simulink model "double_sim_motor"  (R2022b)
settings: Solver=FixedStepAuto  StartTime=0.0  StopTime=T-0.1  RelTol=1e-3
values from neighbouring files (symbols this model uses):
  dt = 0.005    [double_main.m]    (also in double_main_px4.m; double_main_so3.m; se3controller.m = 0.001)
  f1234tofm = [1 1 1 1 ... (first row only)    [double_main.m]    (also in double_main_px4.m; double_main_so3.m; my_exp1.m)
  fmtof1234 = inv(f1234tofm)    [double_main.m]    (also in double_main_px4.m; double_main_so3.m; my_exp1.m)
  J = diag([0.0024 0.0025 0.0041])    [double_main.m]    (also in double_main_px4.m = diag([0.0031 0.0032 0.0045]); double_main_so3.m = diag([0.0031 0.0032 0.0045]); my_exp1.m = diag([Ixx,Iyy,Izz]))
  K = lqr(sys,Q,R)    [double_main.m]    (also in double_main_px4.m; double_main_so3.m)
  kt = 2.03e-8    (= 2.03e-08)    [double_main.m]    (also in double_main_px4.m; double_main_so3.m)
  kv = m*K(1,4)    [double_main.m]    (also in double_main_px4.m = m*K1(1,4); double_main_so3.m = m*K1(1,4); se3controller.m = 2)
  kx = m*K(1,1)    [double_main.m]    (also in double_main_px4.m = m*K1(1,1); double_main_so3.m = m*K1(1,1); se3controller.m = 3)
  m = 0.8    [double_main.m]    (also in double_main_px4.m = 0.8771; double_main_so3.m = 0.8771; my_exp1.m; run_exp1.m = 0.5)
  tau = 0.01    [double_main.m]    (also in double_main_px4.m; double_main_so3.m)
libraries: shared6dof x1, aerolibutil x1
settings Model: Creator=zzy  LastModifiedBy=zzy
settings DataIOCC: ReturnWorkspaceOutputs=off

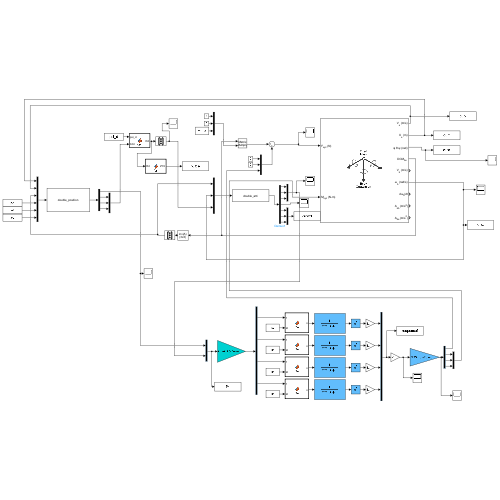
[thumbnail: Simulink's stored preview of the top-level diagram]
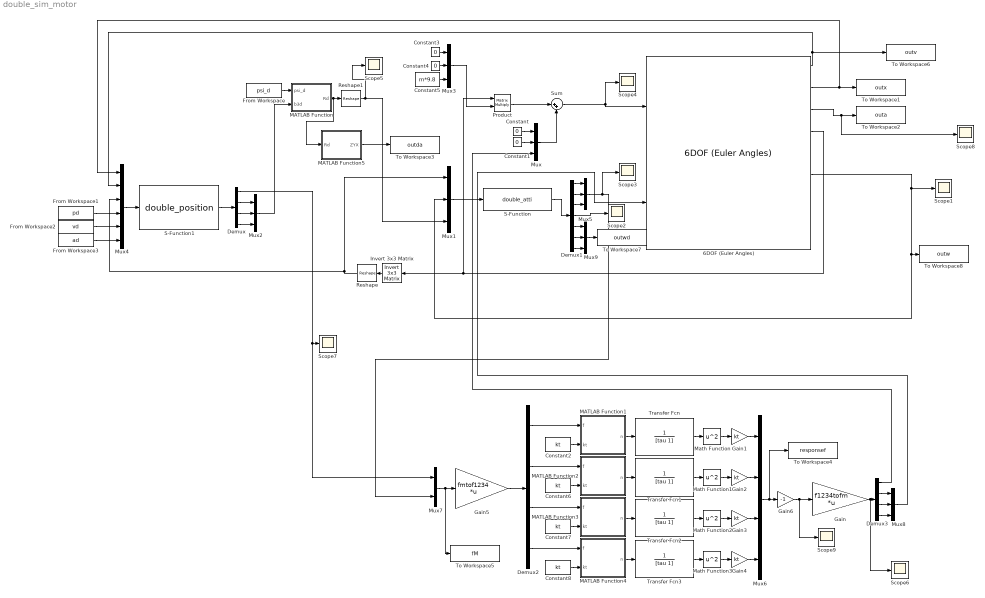
== system double_sim_motor ==
  6DOF (Euler Angles) : shared6dof/6DOF (Euler Angles)  units=Metric (MKS)  mtype=Fixed  rep=Quaternion  xme_0=[0 0 0]  Vm_0=[0 0 0]  eul_0=[0 0 0]  pm_0=[0 0 0]  mass_0=m  mass_e=0.5  mass_f=2.0  inertia=J  inertia_e=eye(3)  inertia_f=2*eye(3)  k_quat=1.0  vre_flag=on  abi_flag=on  aMode=0  xme_statename=''  Vm_statename=''  eul_statename=''  quat_statename=''  pm_statename=''  mass_statename=''
  Constant{,1,3..4} (4 alike) : Constant  Value=0
  Constant{2,6..8} (4 alike) : Constant  Value=kt
  Constant5 : Constant  Value=m*9.8
  Demux : Demux
  Demux1 : Demux  Outputs=7
  Demux2 : Demux
  Demux3 : Demux
  From Workspace : FromWorkspace  VariableName=psi_d
  From Workspace1 : FromWorkspace  VariableName=pd
  From Workspace2 : FromWorkspace  VariableName=vd
  From Workspace3 : FromWorkspace  VariableName=ad
  Gain : Gain  Gain=f1234tofm  Multiplication=Matrix(K*u) (u vector)
  Gain{1..4} (4 alike) : Gain  Gain=kt
  Gain5 : Gain  Gain=fmtof1234  Multiplication=Matrix(K*u) (u vector)
  Gain6 : Gain  Gain=-1
  Invert 3x3 Matrix : aerolibutil/Invert  3x3 Matrix
  MATLAB Function : MATLAB Function  TreatAsAtomicUnit=on
  MATLAB Function1 : MATLAB Function  TreatAsAtomicUnit=on
  MATLAB Function2 : MATLAB Function  TreatAsAtomicUnit=on
  MATLAB Function3 : MATLAB Function  TreatAsAtomicUnit=on
  MATLAB Function4 : MATLAB Function  TreatAsAtomicUnit=on
  MATLAB Function5 : MATLAB Function  TreatAsAtomicUnit=on
  Math Function{,1..3} (4 alike) : Math  Operator=square
  Mux{,1..3,5,8..9} (7 alike) : Mux  Inputs=3
  Mux4 : Mux  Inputs=6
  Mux6 : Mux
  Mux7 : Mux  Inputs=2
  Product : Product  Multiplication=Matrix(*)
  Reshape : Reshape  OutputDimensionality=Column vector (2-D)
  Reshape1 : Reshape  OutputDimensionality=Column vector (2-D)
  S-Function : S-Function  FunctionName=double_atti  Parameters=dt,J,K  SFunctionDeploymentMode=off  EnableBusSupport=off
  S-Function1 : S-Function  FunctionName=double_position  Parameters=dt,m,kx,kv  SFunctionDeploymentMode=off  EnableBusSupport=off
  Scope{1..9} (9 alike) : Scope
  Sum : Sum  Inputs=|++
  To Workspace1 : ToWorkspace  VariableName=outx  SampleTime=-1
      settings: Save2DSignal=2-D array (concatenate along first dimension)
  To Workspace2 : ToWorkspace  VariableName=outa  SampleTime=-1
      settings: Save2DSignal=2-D array (concatenate along first dimension)
  To Workspace3 : ToWorkspace  VariableName=outda  SampleTime=-1
      settings: Save2DSignal=2-D array (concatenate along first dimension)
  To Workspace4 : ToWorkspace  VariableName=responsef  SampleTime=-1
      settings: Save2DSignal=2-D array (concatenate along first dimension)
  To Workspace5 : ToWorkspace  VariableName=fM  SampleTime=-1
      settings: Save2DSignal=2-D array (concatenate along first dimension)
  To Workspace6 : ToWorkspace  VariableName=outv  SampleTime=-1
      settings: Save2DSignal=2-D array (concatenate along first dimension)
  To Workspace7 : ToWorkspace  VariableName=outwd  SampleTime=-1
      settings: Save2DSignal=2-D array (concatenate along first dimension)
  To Workspace8 : ToWorkspace  VariableName=outw  SampleTime=-1
      settings: Save2DSignal=2-D array (concatenate along first dimension)
  Transfer Fcn{,1..3} (4 alike) : TransferFcn  Numerator=1  Denominator=[tau 1]
  wires:
  Constant1/1 -> Mux/2
  Constant/1 -> Mux/1
  6DOF (Euler Angles)/6 -> To Workspace8/1, Mux1/2, Scope1/1
  Invert 3x3 Matrix/1 -> Reshape/1
  Mux1/1 -> S-Function/1
  Reshape/1 -> Mux1/1, Mux4/3
  6DOF (Euler Angles)/3 -> Scope8/1, To Workspace2/1
  From Workspace/1 -> MATLAB Function/1(psi_d)
  MATLAB Function/1(Rd) -> MATLAB Function5/1(Rd), Reshape1/1
  Demux/2 -> Mux2/1
  Demux/4 -> Mux2/3
  Demux/3 -> Mux2/2
  S-Function1/1 -> Demux/1
  Mux2/1 -> MATLAB Function/2(b3d)
  6DOF (Euler Angles)/4 -> Product/1, Invert 3x3 Matrix/1
  Constant3/1 -> Mux3/1
  Mux3/1 -> Product/2
  Constant4/1 -> Mux3/2
  Constant5/1 -> Mux3/3
  Product/1 -> Sum/1
  Mux/1 -> Sum/2
  Sum/1 -> Scope4/1, 6DOF (Euler Angles)/1
  6DOF (Euler Angles)/2 -> To Workspace1/1, Mux4/1
  6DOF (Euler Angles)/1 -> To Workspace6/1, Mux4/2
  From Workspace1/1 -> Mux4/4
  From Workspace2/1 -> Mux4/5
  From Workspace3/1 -> Mux4/6
  Mux4/1 -> S-Function1/1
  Reshape1/1 -> Scope5/1, Mux1/3
  S-Function/1 -> Demux1/1
  Demux1/1 -> Mux5/1
  Demux1/2 -> Mux5/2
  Demux1/3 -> Mux5/3
  Demux1/4 -> Scope2/1
  MATLAB Function1/1(n) -> Transfer Fcn/1
  Constant2/1 -> MATLAB Function1/2(kt)
  Transfer Fcn/1 -> Math Function/1
  Math Function/1 -> Gain1/1
  Constant6/1 -> MATLAB Function2/2(kt)
  Transfer Fcn1/1 -> Math Function1/1
  MATLAB Function2/1(n) -> Transfer Fcn1/1
  Math Function1/1 -> Gain2/1
  Constant7/1 -> MATLAB Function3/2(kt)
  Transfer Fcn2/1 -> Math Function2/1
  MATLAB Function3/1(n) -> Transfer Fcn2/1
  Math Function2/1 -> Gain3/1
  Constant8/1 -> MATLAB Function4/2(kt)
  Transfer Fcn3/1 -> Math Function3/1
  MATLAB Function4/1(n) -> Transfer Fcn3/1
  Math Function3/1 -> Gain4/1
  Demux2/1 -> MATLAB Function1/1(f)
  Demux2/2 -> MATLAB Function2/1(f)
  Demux2/3 -> MATLAB Function3/1(f)
  Demux2/4 -> MATLAB Function4/1(f)
  Gain1/1 -> Mux6/1
  Gain2/1 -> Mux6/2
  Gain3/1 -> Mux6/3
  Gain4/1 -> Mux6/4
  Mux6/1 -> To Workspace4/1, Gain6/1
  Gain5/1 -> Demux2/1
  Mux5/1 -> Scope3/1, Mux7/2
  Mux7/1 -> To Workspace5/1, Gain5/1
  Demux/1 -> Scope7/1, Mux7/1
  Gain/1 -> Scope6/1, Demux3/1
  Demux3/2 -> Mux8/1
  Demux3/3 -> Mux8/2
  Demux3/4 -> Mux8/3
  Mux8/1 -> 6DOF (Euler Angles)/2
  Demux3/1 -> Mux/3
  Gain6/1 -> Scope9/1, Gain/1
  MATLAB Function5/1(ZYX) -> To Workspace3/1
  Demux1/5 -> Mux9/1
  Demux1/6 -> Mux9/2
  Demux1/7 -> Mux9/3
  Mux9/1 -> To Workspace7/1

== matlab function double_sim_motor/MATLAB Function ==
  data: psi_d input; Rd output; b3d input
function Rd = fcn(psi_d,b3d)
b1d=[cos(psi_d);sin(psi_d);0];
b2d=cross(b3d,b1d)/norm(cross(b3d,b1d));
Rd=[cross(b2d,b3d),b2d,b3d];

end

== matlab function double_sim_motor/MATLAB Function2 ==
  data: f input; n output; kt input
function n = f2w(f,kt)
if f<0
    n=sqrt(-f/kt);
else
    n=0;
end

== matlab function double_sim_motor/MATLAB Function3 ==
  data: f input; n output; kt input
function n = f2w(f,kt)
if f<0
    n=sqrt(-f/kt);
else
    n=0;
end

== matlab function double_sim_motor/MATLAB Function4 ==
  data: f input; n output; kt input
function n = f2w(f,kt)
if f<0
    n=sqrt(-f/kt);
else
    n=0;
end

== matlab function double_sim_motor/MATLAB Function5 ==
  data: Rd input; ZYX output
function ZYX = fcn(Rd)
ZYX=rotm2eul(Rd,'ZYX');
end

== matlab function double_sim_motor/MATLAB Function1 ==
  data: f input; n output; kt input
function n = f2w(f,kt)
if f<0
    n=sqrt(-f/kt);
else
    n=0;
end
